simulink model "test_bergeron"  (R2025b)
settings: Solver=FixedStepAuto  StartTime=0.0  StopTime=2  RelTol=1e-3
undefined symbols (not defined in the file): Ts
libraries: ee_lib_for_power_systems x9, ee_lib x6, nesl_utility x3, fl_lib x2
settings Model: Creator=gdudgeon  LastModifiedBy=gdudgeon

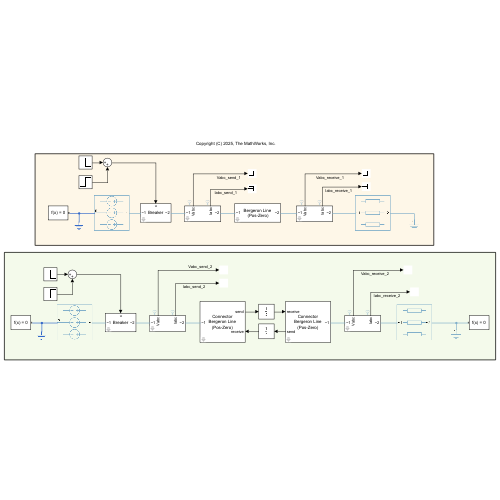
[thumbnail: Simulink's stored preview of the top-level diagram]
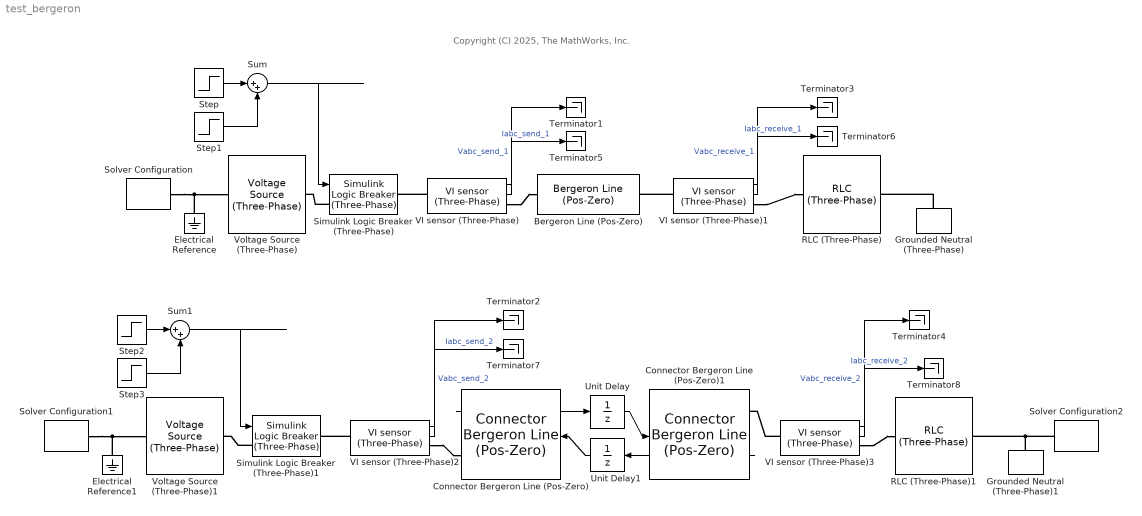
== system test_bergeron ==
  note: Copyright (C) 2025, The MathWorks, Inc.
  Bergeron Line (Pos-Zero) : ee_lib_for_power_systems/Network Components/Bergeron Line (Pos-Zero)  length=100  R1_L1_C1=[0.01 0.001 1e-8]  R0_L0_C0=[0.4 0.004 8e-9]  Ts=5e-5
      settings: SourceProductName=Support Library for Power Systems
  Connector Bergeron Line (Pos-Zero) : ee_lib_for_power_systems/Network Components/Connector Bergeron Line (Pos-Zero)  length=100  R1_L1_C1=[0.01 0.001 1e-8]  R0_L0_C0=[0.4 0.004 8e-9]  Ts=5e-5
      settings: SourceProductName=Support Library for Power Systems
  Connector Bergeron Line (Pos-Zero)1 : ee_lib_for_power_systems/Network Components/Connector Bergeron Line (Pos-Zero)  length=100  R1_L1_C1=[0.01 0.001 1e-8]  R0_L0_C0=[0.4 0.004 8e-9]  Ts=5e-5
      settings: SourceProductName=Support Library for Power Systems
  Electrical Reference : fl_lib/Electrical/Electrical Elements/Electrical Reference
  Electrical Reference1 : fl_lib/Electrical/Electrical Elements/Electrical Reference
  Grounded Neutral (Three-Phase) : ee_lib/Connectors & References/Grounded Neutral (Three-Phase)
  Grounded Neutral (Three-Phase)1 : ee_lib/Connectors & References/Grounded Neutral (Three-Phase)
  RLC (Three-Phase) : ee_lib/Passive/RLC Assemblies/RLC (Three-Phase)  port_option=ee.enum.threePhasePort.composite  component_structure=ee.enum.rlc.structure.SeriesRL  R=1 Ohm  L=1e-3 H  C=1e-6 F  R_parasitic=0 Ohm  G_parasitic=0 1/Ohm  IL_specify=off  IL_priority=High  IL=[0, 0, 0] A  IL_nominal_specify=off  IL_nominal_value=1  IL_nominal_unit=A  VC_specify=off  VC_priority=High  VC=[0, 0, 0] V  VC_nominal_specify=off  VC_nominal_value=1  VC_nominal_unit=V
      settings: InternalSimscapePortConfiguration="{\"Bottom\":[],\"Left\":[{\"id\":\"N1\",\"label\":\"~1\",\"type\":\"foundation.electrical.three_phase\"}],\"Right\":[{\"id\":\"N2\",\"label\":\"~2\",\"type\":\"foundation.electrical.three_phase\"}],\"Top\":[]}"
  RLC (Three-Phase)1 : ee_lib/Passive/RLC Assemblies/RLC (Three-Phase)  port_option=ee.enum.threePhasePort.composite  component_structure=ee.enum.rlc.structure.SeriesRL  R=1 Ohm  L=1e-3 H  C=1e-6 F  R_parasitic=0 Ohm  G_parasitic=0 1/Ohm  IL_specify=off  IL_priority=High  IL=[0, 0, 0] A  IL_nominal_specify=off  IL_nominal_value=1  IL_nominal_unit=A  VC_specify=off  VC_priority=High  VC=[0, 0, 0] V  VC_nominal_specify=off  VC_nominal_value=1  VC_nominal_unit=V
      settings: InternalSimscapePortConfiguration="{\"Bottom\":[],\"Left\":[{\"id\":\"N1\",\"label\":\"~1\",\"type\":\"foundation.electrical.three_phase\"}],\"Right\":[{\"id\":\"N2\",\"label\":\"~2\",\"type\":\"foundation.electrical.three_phase\"}],\"Top\":[]}"
  Simulink Logic Breaker (Three-Phase) : ee_lib_for_power_systems/Network Components/Simulink Logic Breaker (Three-Phase)  initB=1  Ron=1e-6  Goff=1e-6  Ts=5e-5
      settings: SourceProductName=Support Library for Power Systems
  Simulink Logic Breaker (Three-Phase)1 : ee_lib_for_power_systems/Network Components/Simulink Logic Breaker (Three-Phase)  initB=1  Ron=1e-6  Goff=1e-6  Ts=5e-5
      settings: SourceProductName=Support Library for Power Systems
  Solver Configuration : nesl_utility/Solver Configuration  PhysicalDomain=network_engine_domain  SubClassName=solver  LeftPortType=input  RightPortType=generic  Tones=[]  Harmonics=[]  SimulateNoise=off  Profile=off  UseLocalSampling=off  EnableSwitchedLinearOptims=on  FrequencyDomain=off  UseCCode=off  RelTol=0.001  AbsTol=0.001  MinStep=1e-09  ToWorkspace=off  RevertToSquareIcSolve=off  NumHomotopyIterations=100  PhasorMode=off  PhasorModeNumHarmonics=1  ConsistencySolver=NEWTON_XTOL_AFTER_FTOL  IndexReductionMethod=None  DoDC=off  ResidualTolerance=1e-09  ConsistencyTolSource=GLOBAL  ConsistencyAbsTol=0.001  ConsistencyRelTol=0.001  ConsistencyTolFactor=0.001  UseLocalSolver=on  LocalSolverChoice=NE_BACKWARD_EULER_ADVANCER  ResolveIndetEquations=off  FunctionEvalNumThread=1  LocalSolverSampleTime=5e-5  DoFixedCost=off  MaxNonlinIter=1  MaxModeIter=2  ComputeImpulses=off  ImpulseIterations=2  LinearAlgebra=auto  LinearAlgebraNumThread=0  EquationFormulation=NE_TIME_EF  DelaysMemoryBudget=1024  AutomaticFiltering=off  FilteringTimeConstant=0.001  PartitionStorageMethod=AS_NEEDED  PartitionMemoryBudget=1024  PartitionMethod=ROBUST  MultibodyUseLocalSolver=off  MultibodyLocalSolverChoice=ODE1  MultibodyLocalSolverSampleTime=0.001
  Solver Configuration1 : nesl_utility/Solver Configuration  PhysicalDomain=network_engine_domain  SubClassName=solver  LeftPortType=input  RightPortType=generic  Tones=[]  Harmonics=[]  SimulateNoise=off  Profile=off  UseLocalSampling=off  EnableSwitchedLinearOptims=on  FrequencyDomain=off  UseCCode=off  RelTol=0.001  AbsTol=0.001  MinStep=1e-09  ToWorkspace=off  RevertToSquareIcSolve=off  NumHomotopyIterations=100  PhasorMode=off  PhasorModeNumHarmonics=1  ConsistencySolver=NEWTON_XTOL_AFTER_FTOL  IndexReductionMethod=None  DoDC=off  ResidualTolerance=1e-09  ConsistencyTolSource=GLOBAL  ConsistencyAbsTol=0.001  ConsistencyRelTol=0.001  ConsistencyTolFactor=0.001  UseLocalSolver=on  LocalSolverChoice=NE_BACKWARD_EULER_ADVANCER  ResolveIndetEquations=off  FunctionEvalNumThread=1  LocalSolverSampleTime=5e-5  DoFixedCost=off  MaxNonlinIter=1  MaxModeIter=2  ComputeImpulses=off  ImpulseIterations=2  LinearAlgebra=auto  LinearAlgebraNumThread=0  EquationFormulation=NE_TIME_EF  DelaysMemoryBudget=1024  AutomaticFiltering=off  FilteringTimeConstant=0.001  PartitionStorageMethod=AS_NEEDED  PartitionMemoryBudget=1024  PartitionMethod=ROBUST  MultibodyUseLocalSolver=off  MultibodyLocalSolverChoice=ODE1  MultibodyLocalSolverSampleTime=0.001
  Solver Configuration2 : nesl_utility/Solver Configuration  PhysicalDomain=network_engine_domain  SubClassName=solver  LeftPortType=input  RightPortType=generic  Tones=[]  Harmonics=[]  SimulateNoise=off  Profile=off  UseLocalSampling=off  EnableSwitchedLinearOptims=on  FrequencyDomain=off  UseCCode=off  RelTol=0.001  AbsTol=0.001  MinStep=1e-09  ToWorkspace=off  RevertToSquareIcSolve=off  NumHomotopyIterations=100  PhasorMode=off  PhasorModeNumHarmonics=1  ConsistencySolver=NEWTON_XTOL_AFTER_FTOL  IndexReductionMethod=None  DoDC=off  ResidualTolerance=1e-09  ConsistencyTolSource=GLOBAL  ConsistencyAbsTol=0.001  ConsistencyRelTol=0.001  ConsistencyTolFactor=0.001  UseLocalSolver=on  LocalSolverChoice=NE_BACKWARD_EULER_ADVANCER  ResolveIndetEquations=off  FunctionEvalNumThread=1  LocalSolverSampleTime=5e-5  DoFixedCost=off  MaxNonlinIter=1  MaxModeIter=2  ComputeImpulses=off  ImpulseIterations=2  LinearAlgebra=auto  LinearAlgebraNumThread=0  EquationFormulation=NE_TIME_EF  DelaysMemoryBudget=1024  AutomaticFiltering=off  FilteringTimeConstant=0.001  PartitionStorageMethod=AS_NEEDED  PartitionMemoryBudget=1024  PartitionMethod=ROBUST  MultibodyUseLocalSolver=off  MultibodyLocalSolverChoice=ODE1  MultibodyLocalSolverSampleTime=0.001
  Step : Step  Before=1  After=0  SampleTime=0
  Step1 : Step  Time=1+1.3/60  SampleTime=0
  Step2 : Step  Before=1  After=0  SampleTime=0
  Step3 : Step  Time=1+1.3/60  SampleTime=0
  Sum : Sum  Inputs=|++
  Sum1 : Sum  Inputs=|++
  Terminator{1..8} (8 alike) : Terminator
  Unit Delay : UnitDelay  SampleTime=Ts  HasFrameUpgradeWarning=on
  Unit Delay1 : UnitDelay  SampleTime=Ts  HasFrameUpgradeWarning=on
  VI sensor (Three-Phase){,1..3} (4 alike) : ee_lib_for_power_systems/Sense and Measure/VI sensor (Three-Phase)  volt_meas=Phase-to-Ground (Phase Voltage)  meas_units=SI  Vnom=24e3  Pnom=100e6
      settings: SourceProductName=Support Library for Power Systems
  Voltage Source (Three-Phase) : ee_lib/Sources/Voltage Source (Three-Phase)  vline_rms=100 V  shift=0 deg  freq=60 Hz  impedance_option=0  SShortCircuit=1e6 A*V  XR=15  R=0.01 Ohm  L=3.97e-4 H  harmonic_option=0  harmonic_orders=[5, 7, 11, 13]  harmonic_ratios=[.1, .1, .1, .1]  G_parasitic=0 1/Ohm  I_specify=off  I_priority=None  I=[0, 0, 0] A  I_nominal_specify=off  I_nominal_value=1  I_nominal_unit=A
  Voltage Source (Three-Phase)1 : ee_lib/Sources/Voltage Source (Three-Phase)  vline_rms=100 V  shift=0 deg  freq=60 Hz  impedance_option=0  SShortCircuit=1e6 A*V  XR=15  R=0.01 Ohm  L=3.97e-4 H  harmonic_option=0  harmonic_orders=[5, 7, 11, 13]  harmonic_ratios=[.1, .1, .1, .1]  G_parasitic=0 1/Ohm  I_specify=off  I_priority=None  I=[0, 0, 0] A  I_nominal_specify=off  I_nominal_value=1  I_nominal_unit=A
  wires:
  Step/1 -> Sum/1
  Step1/1 -> Sum/2
  Sum/1 -> Simulink Logic Breaker (Three-Phase)/1
  VI sensor (Three-Phase)/1 -> Terminator1/1  "Vabc_send_1"
  VI sensor (Three-Phase)1/1 -> Terminator3/1  "Vabc_receive_1"
  VI sensor (Three-Phase)/2 -> Terminator5/1  "Iabc_send_1"
  VI sensor (Three-Phase)1/2 -> Terminator6/1  "Iabc_receive_1"
  VI sensor (Three-Phase)3/2 -> Terminator8/1  "Iabc_receive_2"
  VI sensor (Three-Phase)2/2 -> Terminator7/1  "Iabc_send_2"
  VI sensor (Three-Phase)3/1 -> Terminator4/1  "Vabc_receive_2"
  VI sensor (Three-Phase)2/1 -> Terminator2/1  "Vabc_send_2"
  Connector Bergeron Line (Pos-Zero)/1 -> Unit Delay/1
  Unit Delay/1 -> Connector Bergeron Line (Pos-Zero)1/1
  Connector Bergeron Line (Pos-Zero)1/1 -> Unit Delay1/1
  Unit Delay1/1 -> Connector Bergeron Line (Pos-Zero)/1
  Sum1/1 -> Simulink Logic Breaker (Three-Phase)1/1
  Step3/1 -> Sum1/2
  Step2/1 -> Sum1/1
  connections:
  Electrical Reference/LConn1 -- Voltage Source (Three-Phase)/LConn1 -- Solver Configuration/RConn1
  Grounded Neutral (Three-Phase)/LConn1 -- RLC (Three-Phase)/RConn1
  Simulink Logic Breaker (Three-Phase)/LConn1 -- Voltage Source (Three-Phase)/RConn1
  VI sensor (Three-Phase)/LConn1 -- Simulink Logic Breaker (Three-Phase)/RConn1
  VI sensor (Three-Phase)/RConn1 -- Bergeron Line (Pos-Zero)/LConn1
  VI sensor (Three-Phase)1/LConn1 -- Bergeron Line (Pos-Zero)/RConn1
  Electrical Reference1/LConn1 -- Solver Configuration1/RConn1 -- Voltage Source (Three-Phase)1/LConn1
  VI sensor (Three-Phase)3/RConn1 -- RLC (Three-Phase)1/LConn1
  VI sensor (Three-Phase)2/RConn1 -- Connector Bergeron Line (Pos-Zero)/RConn1
  Simulink Logic Breaker (Three-Phase)1/LConn1 -- Voltage Source (Three-Phase)1/RConn1
  VI sensor (Three-Phase)3/LConn1 -- Connector Bergeron Line (Pos-Zero)1/RConn1
  Grounded Neutral (Three-Phase)1/LConn1 -- RLC (Three-Phase)1/RConn1 -- Solver Configuration2/RConn1
  VI sensor (Three-Phase)1/RConn1 -- RLC (Three-Phase)/LConn1
  VI sensor (Three-Phase)2/LConn1 -- Simulink Logic Breaker (Three-Phase)1/RConn1
